simulink library "magnetorquer_assembly_lib"  (R2016b)
settings: Solver=VariableStepAuto  StartTime=0.0  StopTime=10.0  RelTol=1e-3
undefined symbols (not defined in the file or in its folder): fsw_params, sim_params
libraries: simulink x6
settings Model: Creator=taylorreynolds  LastModifiedBy=Taylor

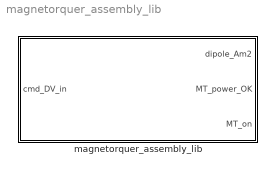
== system magnetorquer_assembly_lib ==
  magnetorquer_assembly_lib : Subsystem

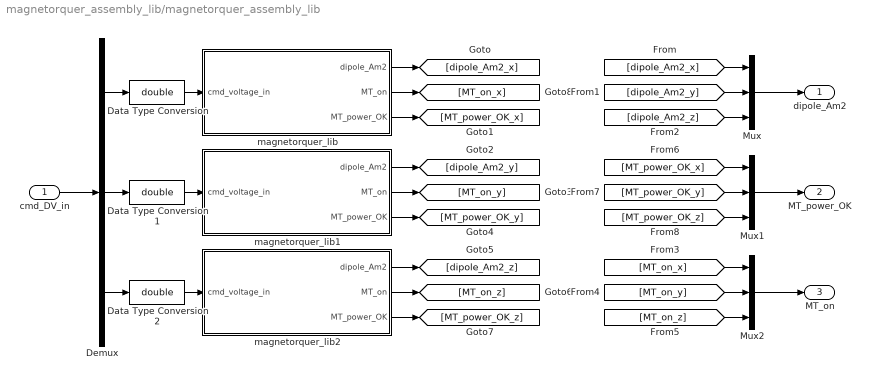
== system magnetorquer_assembly_lib/magnetorquer_assembly_lib ==
  cmd_DV_in : Inport
  Data Type Conversion : DataTypeConversion  OutDataTypeStr=double  RndMeth=Nearest
  Data Type Conversion1 : DataTypeConversion  OutDataTypeStr=double  RndMeth=Nearest
  Data Type Conversion2 : DataTypeConversion  OutDataTypeStr=double  RndMeth=Nearest
  Demux : Demux  Outputs=3
  Mux : Mux  Inputs=3
  Mux1 : Mux  Inputs=[1 1 1]
  Mux2 : Mux  Inputs=[1 1 1]
  magnetorquer_lib : Subsystem  mask{voltage_to_dipole=fsw_params.control.cmd_processing.dv_2_m_X, upperbound=sim_params.actuators.magnetorquer.max_dipole_x, lowerbound=-sim_params.actuators.magnetorquer.max_dipole_x}
      mask prompts: voltage_to_dipole "Simulink:blkprm_prompts:GainGain"; upperbound "Simulink:masks:UpperBound_MP"; lowerbound "Simulink:masks:LowerBound_MP"
      mask TypeOptions voltage_to_dipole: Gain/Gain
      mask TypeOptions upperbound:
      | Check
      | Static Range/max
      mask TypeOptions lowerbound:
      | Check
      | Static Range/min
  magnetorquer_lib1 : Subsystem  mask{voltage_to_dipole=fsw_params.control.cmd_processing.dv_2_m_Y, upperbound=sim_params.actuators.magnetorquer.max_dipole_y, lowerbound=-sim_params.actuators.magnetorquer.max_dipole_y}
      mask prompts: voltage_to_dipole "Simulink:blkprm_prompts:GainGain"; upperbound "Simulink:masks:UpperBound_MP"; lowerbound "Simulink:masks:LowerBound_MP"
      mask TypeOptions voltage_to_dipole: Gain/Gain
      mask TypeOptions upperbound:
      | Check
      | Static Range/max
      mask TypeOptions lowerbound:
      | Check
      | Static Range/min
  magnetorquer_lib2 : Subsystem  mask{voltage_to_dipole=fsw_params.control.cmd_processing.dv_2_m_Z, upperbound=sim_params.actuators.magnetorquer.max_dipole_z, lowerbound=-sim_params.actuators.magnetorquer.max_dipole_z}
      mask prompts: voltage_to_dipole "Simulink:blkprm_prompts:GainGain"; upperbound "Simulink:masks:UpperBound_MP"; lowerbound "Simulink:masks:LowerBound_MP"
      mask TypeOptions voltage_to_dipole: Gain/Gain
      mask TypeOptions upperbound:
      | Check
      | Static Range/max
      mask TypeOptions lowerbound:
      | Check
      | Static Range/min
  dipole_Am2 : Outport
  MT_power_OK : Outport  Port=2
  MT_on : Outport  Port=3
  wires:
  cmd_DV_in/1 -> Demux/1
  Demux/3 -> Data Type Conversion2/1
  Demux/1 -> Data Type Conversion/1
  Demux/2 -> Data Type Conversion1/1
  magnetorquer_lib/1(dipole_Am2) -> [dipole_Am2_x]
  magnetorquer_lib2/3(MT_power_OK) -> [MT_power_OK_z]
  magnetorquer_lib2/2(MT_on) -> [MT_on_z]
  magnetorquer_lib2/1(dipole_Am2) -> [dipole_Am2_z]
  magnetorquer_lib1/3(MT_power_OK) -> [MT_power_OK_y]
  magnetorquer_lib1/2(MT_on) -> [MT_on_y]
  magnetorquer_lib1/1(dipole_Am2) -> [dipole_Am2_y]
  magnetorquer_lib/3(MT_power_OK) -> [MT_power_OK_x]
  magnetorquer_lib/2(MT_on) -> [MT_on_x]
  Mux/1 -> dipole_Am2/1
  [dipole_Am2_x] -> Mux/1
  [dipole_Am2_y] -> Mux/2
  [dipole_Am2_z] -> Mux/3
  [MT_on_x] -> Mux2/1
  [MT_on_y] -> Mux2/2
  [MT_on_z] -> Mux2/3
  [MT_power_OK_x] -> Mux1/1
  [MT_power_OK_y] -> Mux1/2
  [MT_power_OK_z] -> Mux1/3
  Mux1/1 -> MT_power_OK/1
  Mux2/1 -> MT_on/1
  Data Type Conversion/1 -> magnetorquer_lib/1(cmd_voltage_in)
  Data Type Conversion1/1 -> magnetorquer_lib1/1(cmd_voltage_in)
  Data Type Conversion2/1 -> magnetorquer_lib2/1(cmd_voltage_in)

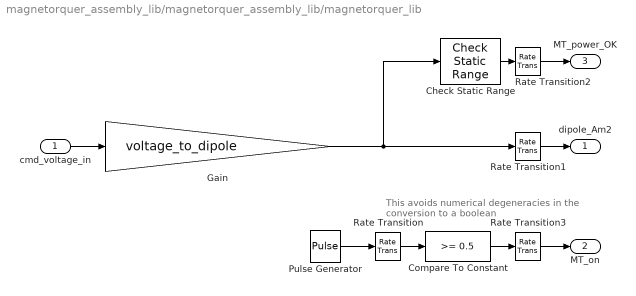
== system magnetorquer_assembly_lib/magnetorquer_assembly_lib/magnetorquer_lib ==
  note: This avoids numerical degeneracies in
      | the conversion to a boolean
  cmd_voltage_in : Inport
  Check Static Range : simulink/Model Verification/Check  Static Range  Description=lowerbound <= u <= upperbound  max=upperbound  max_included=on  min=lowerbound  min_included=on  enabled=on  stopWhenAssertionFail=off  export=on  icon=graphic
  Compare To Constant : simulink/Logic and Bit Operations/Compare To Constant  relop=>=  const=0.5  OutDataTypeStr=boolean
  Gain : Gain  Gain=voltage_to_dipole
  Pulse Generator : DiscretePulseGenerator  PulseType=Time based  Period=sim_params.CAN.sync_pulse_s  PulseWidth=fsw_params.actuators.pct_sync_pulse
  Rate Transition{,1..3} (4 alike) : RateTransition
  dipole_Am2 : Outport
  MT_on : Outport  Port=2
  MT_power_OK : Outport  Port=3
  wires:
  Check Static Range/1 -> Rate Transition2/1
  Pulse Generator/1 -> Rate Transition/1
  Gain/1 -> Rate Transition1/1, Check Static Range/1
  cmd_voltage_in/1 -> Gain/1
  Compare To Constant/1 -> Rate Transition3/1
  Rate Transition/1 -> Compare To Constant/1
  Rate Transition1/1 -> dipole_Am2/1
  Rate Transition2/1 -> MT_power_OK/1
  Rate Transition3/1 -> MT_on/1

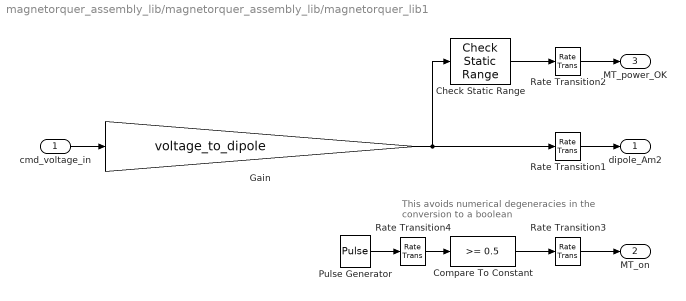
== system magnetorquer_assembly_lib/magnetorquer_assembly_lib/magnetorquer_lib1 ==
  note: This avoids numerical degeneracies in
      | the conversion to a boolean
  cmd_voltage_in : Inport
  Check Static Range : simulink/Model Verification/Check  Static Range  Description=lowerbound <= u <= upperbound  max=upperbound  max_included=on  min=lowerbound  min_included=on  enabled=on  stopWhenAssertionFail=off  export=on  icon=graphic
  Compare To Constant : simulink/Logic and Bit Operations/Compare To Constant  relop=>=  const=0.5  OutDataTypeStr=boolean
  Gain : Gain  Gain=voltage_to_dipole
  Pulse Generator : DiscretePulseGenerator  PulseType=Time based  Period=sim_params.CAN.sync_pulse_s  PulseWidth=fsw_params.actuators.pct_sync_pulse
  Rate Transition{1..4} (4 alike) : RateTransition
  dipole_Am2 : Outport
  MT_on : Outport  Port=2
  MT_power_OK : Outport  Port=3
  wires:
  Check Static Range/1 -> Rate Transition2/1
  Gain/1 -> Rate Transition1/1, Check Static Range/1
  cmd_voltage_in/1 -> Gain/1
  Pulse Generator/1 -> Rate Transition4/1
  Compare To Constant/1 -> Rate Transition3/1
  Rate Transition2/1 -> MT_power_OK/1
  Rate Transition1/1 -> dipole_Am2/1
  Rate Transition3/1 -> MT_on/1
  Rate Transition4/1 -> Compare To Constant/1

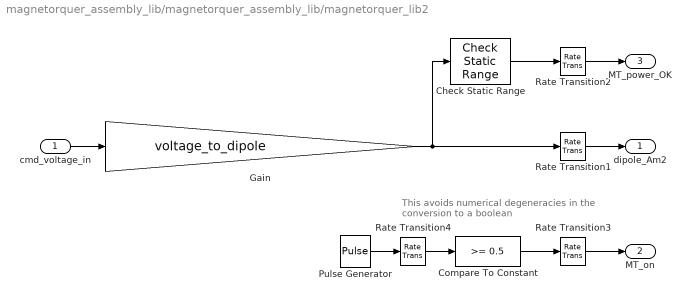
== system magnetorquer_assembly_lib/magnetorquer_assembly_lib/magnetorquer_lib2 ==
  note: This avoids numerical degeneracies in
      | the conversion to a boolean
  cmd_voltage_in : Inport
  Check Static Range : simulink/Model Verification/Check  Static Range  Description=lowerbound <= u <= upperbound  max=upperbound  max_included=on  min=lowerbound  min_included=on  enabled=on  stopWhenAssertionFail=off  export=on  icon=graphic
  Compare To Constant : simulink/Logic and Bit Operations/Compare To Constant  relop=>=  const=0.5  OutDataTypeStr=boolean
  Gain : Gain  Gain=voltage_to_dipole
  Pulse Generator : DiscretePulseGenerator  PulseType=Time based  Period=sim_params.CAN.sync_pulse_s  PulseWidth=fsw_params.actuators.pct_sync_pulse
  Rate Transition{1..4} (4 alike) : RateTransition
  dipole_Am2 : Outport
  MT_on : Outport  Port=2
  MT_power_OK : Outport  Port=3
  wires:
  Check Static Range/1 -> Rate Transition2/1
  Gain/1 -> Rate Transition1/1, Check Static Range/1
  cmd_voltage_in/1 -> Gain/1
  Pulse Generator/1 -> Rate Transition4/1
  Compare To Constant/1 -> Rate Transition3/1
  Rate Transition2/1 -> MT_power_OK/1
  Rate Transition1/1 -> dipole_Am2/1
  Rate Transition3/1 -> MT_on/1
  Rate Transition4/1 -> Compare To Constant/1
